simulink library "commdigpbndpm2"  (Simulink 5.0)
undefined symbols (not defined in the file or in its folder): D
libraries: commblksprivate x12, dspsigattribs x6, commdigbbndpm2 x6, dspsigops x3
settings Model: RequirementInfo=9  CovMetricSettings=d  Creator=tdelve  LastModifiedBy=mmclerno

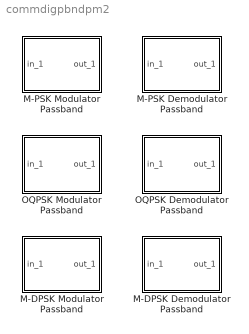
== system commdigpbndpm2 ==
  M-DPSK Demodulator Passband : Subsystem  mask(M-DPSK Demodulator Passband){M=8, OutType=Integer, Dec=Binary, td=1/100, numSamp=1, Fc=3000, Ph=pi/8, InSamp=1/8000}
      mask prompts: M "M-ary number:"; OutType "Output type:"; Dec "Constellation ordering:"; td "Symbol periodl (s):"; numSamp "Baseband samples per symbol:"; Fc "Carrier frequency (Hz):"; Ph "Carrier initial phase (rad):"; InSamp "Input sample time (s):"
      mask help:
      | Demodulate the input signal using the differential phase shift keying method.
      |
      | The input signal must be a sample-based scalar. In case of bit output, the width of the output is the number of bits per symbol. The symbols can be either binary-demapped or Gray-demapped into bits.
      mask init:
      | commblkdyampmdemod('M-DPSK Demodulator Baseband','update');
      | commblkpbndpskmod(gcb,'init');
      mask Help: helpview(commbhelp)
      mask StyleString: edit,popup(Bit|Integer),popup(Binary|Gray),edit,edit,edit,edit,edit
      mask CallbackString: |commblkpbndpskmod(gcb,'InType');||||||
      mask Display:
      | plot(0,0,100,100,[5+1.5*[[0:.8:10] [10:1.6:20] [20:.8:30]] 50 50 50 50+15*[0 1 1 2 2 3]],[85+10*[sin([0:.8:10]*pi*2/5) sin([10:1.6:20]*pi/5) sin([20:.8:30]*pi*2/5)] 85 99 75 85+8*[1 1 -1 -1 1 1]]);
      | disp('M-DPSK')
  M-DPSK Modulator Passband : Subsystem  mask(M-DPSK Modulator Passband){M=8, InType=Integer, Enc=Binary, td=1/100, numSamp=1, Fc=3000, Ph=pi/8, OutSamp=1/8000}
      mask prompts: M "M-ary number:"; InType "Input type:"; Enc "Constellation ordering:"; td "Symbol period (s):"; numSamp "Baseband samples per symbol:"; Fc "Carrier frequency (Hz):"; Ph "Carrier initial phase (rad):"; OutSamp "Output sample time (s):"
      mask help:
      | Modulate the input signal using the differential phase shift keying method.
      |
      | The input signal must be sample-based. In case of integer input, the input must be a scalar. In case of bit input, the width of the input must equal the number of bits per symbol. The bits can be either binary-mapped or Gray-mapped into symbols.
      |
      | The input sample time must equal the symbol period.
      mask init:
      | commblkdyampmmod('M-DPSK Modulator Baseband','update');
      | commblkpbndpskmod(gcb,'init');
      mask Help: helpview(commbhelp)
      mask StyleString: edit,popup(Bit|Integer),popup(Binary|Gray),edit,edit,edit,edit,edit
      mask CallbackString: |commblkpbndpskmod(gcb,'InType');||||||
      mask Display:
      | plot(0,0,100,100,[5+15*[0 1 1 2 2 3] 50 50 50 50+1.5*[[0:.8:10] [10:1.6:20] [20:.8:30]]],[85+8*[1 1 -1 -1 1 1] 85 99 75 85+10*[sin([0:.8:10]*pi*2/5) sin([10:1.6:20]*pi/5) sin([20:.8:30]*pi*2/5)]]);
      | disp('M-DPSK')
  M-PSK Demodulator Passband : Subsystem  mask(M-PSK Demodulator Passband){M=8, OutType=Integer, Dec=Binary, td=1/100, numSamp=1, Fc=3000, Ph=pi/8, InSamp=1/8000}
      mask prompts: M "M-ary number:"; OutType "Output type:"; Dec "Constellation ordering:"; td "Symbol period (s):"; numSamp "Baseband samples per symbol:"; Fc "Carrier frequency (Hz):"; Ph "Carrier initial phase (rad):"; InSamp "Input sample time (s):"
      mask help:
      | Demodulate the input signal using the phase shift keying method.
      |
      | The input signal must be a sample-based scalar. In case of bit output, the width of the output is the number of bits per symbol. The symbols can be either binary-demapped or Gray-demapped into bits.
      mask init:
      | commblkdyampmdemod('M-PSK Demodulator Baseband','update');
      | commblkpbndpskmod(gcb,'init');
      mask Help: helpview(commbhelp)
      mask StyleString: edit,popup(Bit|Integer),popup(Binary|Gray),edit,edit,edit,edit,edit
      mask CallbackString: |commblkpbndpskmod(gcb,'InType');||||||
      mask Display:
      | plot(0,0,100,100,[5+1.5*[[0:.8:10] [10:1.6:20] [20:.8:30]] 50 50 50 50+15*[0 1 1 2 2 3]],[85+10*[sin([0:.8:10]*pi*2/5) sin([10:1.6:20]*pi/5) sin([20:.8:30]*pi*2/5)] 85 99 75 85+8*[1 1 -1 -1 1 1]]);
      | disp('M-PSK')
  M-PSK Modulator Passband : Subsystem  mask(M-PSK Modulator Passband){M=8, InType=Integer, Enc=Binary, td=1/100, numSamp=1, Fc=3000, Ph=pi/8, OutSamp=1/8000}
      mask prompts: M "M-ary number:"; InType "Input type:"; Enc "Constellation ordering:"; td "Symbol period (s):"; numSamp "Baseband samples per symbol:"; Fc "Carrier frequency (Hz):"; Ph "Carrier initial phase (rad):"; OutSamp "Output sample time (s):"
      mask help:
      | Modulate the input signal using the phase shift keying method.
      |
      | The input signal must be sample-based. In case of integer input, the input must be a scalar. In case of bit input, the width of the input must equal the number of bits per symbol. The bits can be either binary-mapped or Gray-mapped into symbols.
      |
      | The input sample time must equal the symbol period.
      mask init:
      | commblkdyampmmod('M-PSK Modulator Baseband','update');
      | commblkpbndpskmod(gcb,'init');
      mask Help: helpview(commbhelp)
      mask StyleString: edit,popup(Bit|Integer),popup(Binary|Gray),edit,edit,edit,edit,edit
      mask CallbackString: |commblkpbndpskmod(gcb,'InType');||||||
      mask Display:
      | plot(0,0,100,100,[5+15*[0 1 1 2 2 3] 50 50 50 50+1.5*[[0:.8:10] [10:1.6:20] [20:.8:30]]],[85+8*[1 1 -1 -1 1 1] 85 99 75 85+10*[sin([0:.8:10]*pi*2/5) sin([10:1.6:20]*pi/5) sin([20:.8:30]*pi*2/5)]]);
      | disp('M-PSK')
  OQPSK Demodulator Passband : Subsystem  mask(OQPSK Demodulator Passband){OutType=Integer, td=1/100, numSamp=7, Fc=3000, Ph=0, InSamp=1/10000}
      mask prompts: OutType "Output type:"; td "Symbol period (s):"; numSamp "Baseband samples per symbol:"; Fc "Carrier frequency (Hz):"; Ph "Carrier initial phase (rad):"; InSamp "Input sample time (s):"
      mask help:
      | Demodulate an offset quadrature phase shift keying modulated signal.
      |
      | The input signal must be a sample-based scalar. In case of bit output, the width of the output is two.
      mask init:
      | commblkdyampmdemod('OQPSK Demodulator Baseband','update');
      mask Help: helpview(commbhelp)
      mask StyleString: popup(Bit|Integer),edit,edit,edit,edit,edit
      mask Display:
      | plot(0,0,100,100,[5+1.5*[[0:.8:10] [10:1.6:20] [20:.8:30]] 50 50 50 50+15*[0 1 1 2 2 3]],[85+10*[sin([0:.8:10]*pi*2/5) sin([10:1.6:20]*pi/5) sin([20:.8:30]*pi*2/5)] 85 99 75 85+8*[1 1 -1 -1 1 1]]);
      | disp('OQPSK')
  OQPSK Modulator Passband : Subsystem  mask(OQPSK Modulator Passband){InType=Integer, td=1/100, numSamp=7, Fc=3000, Ph=0, OutSamp=1/10000}
      mask prompts: InType "Input type:"; td "Symbol period (s):"; numSamp "Baseband samples per symbol:"; Fc "Carrier frequency (Hz):"; Ph "Carrier initial phase (rad):"; OutSamp "Output sample time (s):"
      mask help:
      | Modulate the input signal using offset quadrature phase shift keying method.
      |
      | The input signal must be sample-based. In case of integer input, the input must be a scalar. In case of bit input, the width of the input must be two.
      |
      | The input sample time must equal the symbol period.
      mask init:
      | commblkdyampmmod('OQPSK Modulator Baseband','update');
      mask Help: helpview(commbhelp)
      mask StyleString: popup(Bit|Integer),edit,edit,edit,edit,edit
      mask Display:
      | plot(0,0,100,100,[5+15*[0 1 1 2 2 3] 50 50 50 50+1.5*[[0:.8:10] [10:1.6:20] [20:.8:30]]],[85+8*[1 1 -1 -1 1 1] 85 99 75 85+10*[sin([0:.8:10]*pi*2/5) sin([10:1.6:20]*pi/5) sin([20:.8:30]*pi*2/5)]]);
      | disp('OQPSK')

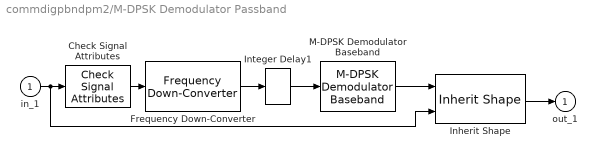
== system commdigpbndpm2/M-DPSK Demodulator Passband ==
  in_1 : Inport
  Check Signal Attributes : dspsigattribs/Check Signal Attributes  SigAttribCheckMethod=Matches attributes exactly  Complexity=Ignore  Frame=Frame-based  DimsCheckMethod=Ignore  Dimensions=1-D  DatatypeCheckMethod=Ignore  DatatypeGeneral=Boolean  DtypeFloatSpecific=Any floating-point  DtypeFixedSpecific=Any fixed-point  DtypeIntSpecific=Any integer  SampleMode=Ignore
  Frequency Down-Converter : commblksprivate/Frequency Down-Converter  Fc=Fc  Ph=Ph  Tin=InSamp  Tout=td/numSamp
  Inherit Shape : commblksprivate/Inherit Shape
  Integer Delay1 : dspsigops/Integer Delay  delay=numSamp-1  ic=0
  M-DPSK Demodulator Baseband : commdigbbndpm2/M-DPSK Demodulator Baseband  M=M  OutType=Integer  Dec=Binary  Ph=0  numSamp=numSamp
  out_1 : Outport  InitialOutput=0
  wires:
  in_1/1 -> Check Signal Attributes/1, Inherit Shape/2
  Check Signal Attributes/1 -> Frequency Down-Converter/1
  Frequency Down-Converter/1 -> Integer Delay1/1
  Integer Delay1/1 -> M-DPSK Demodulator Baseband/1
  M-DPSK Demodulator Baseband/1 -> Inherit Shape/1
  Inherit Shape/1 -> out_1/1

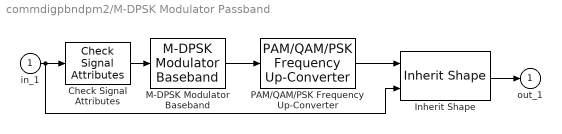
== system commdigpbndpm2/M-DPSK Modulator Passband ==
  in_1 : Inport
  Check Signal Attributes : dspsigattribs/Check Signal Attributes  SigAttribCheckMethod=Matches attributes exactly  Complexity=Ignore  Frame=Frame-based  DimsCheckMethod=Ignore  Dimensions=1-D  DatatypeCheckMethod=Ignore  DatatypeGeneral=Boolean  DtypeFloatSpecific=Any floating-point  DtypeFixedSpecific=Any fixed-point  DtypeIntSpecific=Any integer  SampleMode=Ignore
  Inherit Shape : commblksprivate/Inherit Shape
  M-DPSK Modulator Baseband : commdigbbndpm2/M-DPSK Modulator Baseband  M=M  InType=Integer  Enc=Binary  Ph=0  numSamp=numSamp
  PAM/QAM/PSK Frequency Up-Converter : commblksprivate/PAM//QAM//PSK Frequency Up-Converter  Fc=Fc  Ph=Ph  Tin=td/numSamp  Tout=OutSamp
  out_1 : Outport  InitialOutput=0
  wires:
  in_1/1 -> Check Signal Attributes/1, Inherit Shape/2
  Check Signal Attributes/1 -> M-DPSK Modulator Baseband/1
  M-DPSK Modulator Baseband/1 -> PAM/QAM/PSK Frequency Up-Converter/1
  PAM/QAM/PSK Frequency Up-Converter/1 -> Inherit Shape/1
  Inherit Shape/1 -> out_1/1

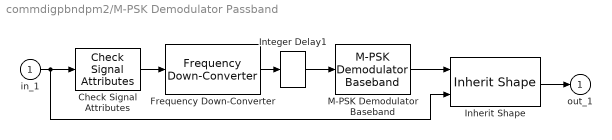
== system commdigpbndpm2/M-PSK Demodulator Passband ==
  in_1 : Inport
  Check Signal Attributes : dspsigattribs/Check Signal Attributes  SigAttribCheckMethod=Matches attributes exactly  Complexity=Ignore  Frame=Frame-based  DimsCheckMethod=Ignore  Dimensions=1-D  DatatypeCheckMethod=Ignore  DatatypeGeneral=Boolean  DtypeFloatSpecific=Any floating-point  DtypeFixedSpecific=Any fixed-point  DtypeIntSpecific=Any integer  SampleMode=Ignore
  Frequency Down-Converter : commblksprivate/Frequency Down-Converter  Fc=Fc  Ph=Ph  Tin=InSamp  Tout=td/numSamp
  Inherit Shape : commblksprivate/Inherit Shape
  Integer Delay1 : dspsigops/Integer Delay  delay=numSamp-1  ic=0
  M-PSK Demodulator Baseband : commdigbbndpm2/M-PSK Demodulator Baseband  M=M  OutType=Integer  Dec=Binary  Ph=0  numSamp=numSamp
  out_1 : Outport  InitialOutput=0
  wires:
  in_1/1 -> Check Signal Attributes/1, Inherit Shape/2
  Check Signal Attributes/1 -> Frequency Down-Converter/1
  Frequency Down-Converter/1 -> Integer Delay1/1
  Integer Delay1/1 -> M-PSK Demodulator Baseband/1
  M-PSK Demodulator Baseband/1 -> Inherit Shape/1
  Inherit Shape/1 -> out_1/1

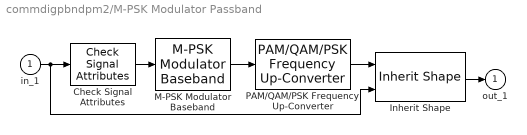
== system commdigpbndpm2/M-PSK Modulator Passband ==
  in_1 : Inport
  Check Signal Attributes : dspsigattribs/Check Signal Attributes  SigAttribCheckMethod=Matches attributes exactly  Complexity=Ignore  Frame=Frame-based  DimsCheckMethod=Ignore  Dimensions=1-D  DatatypeCheckMethod=Ignore  DatatypeGeneral=Boolean  DtypeFloatSpecific=Any floating-point  DtypeFixedSpecific=Any fixed-point  DtypeIntSpecific=Any integer  SampleMode=Ignore
  Inherit Shape : commblksprivate/Inherit Shape
  M-PSK Modulator Baseband : commdigbbndpm2/M-PSK Modulator Baseband  M=M  InType=Integer  Enc=Binary  Ph=0  numSamp=numSamp
  PAM/QAM/PSK Frequency Up-Converter : commblksprivate/PAM//QAM//PSK Frequency Up-Converter  Fc=Fc  Ph=Ph  Tin=td/numSamp  Tout=OutSamp
  out_1 : Outport  InitialOutput=0
  wires:
  in_1/1 -> Inherit Shape/2, Check Signal Attributes/1
  Check Signal Attributes/1 -> M-PSK Modulator Baseband/1
  M-PSK Modulator Baseband/1 -> PAM/QAM/PSK Frequency Up-Converter/1
  PAM/QAM/PSK Frequency Up-Converter/1 -> Inherit Shape/1
  Inherit Shape/1 -> out_1/1

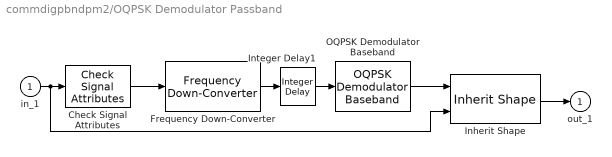
== system commdigpbndpm2/OQPSK Demodulator Passband ==
  in_1 : Inport
  Check Signal Attributes : dspsigattribs/Check Signal Attributes  SigAttribCheckMethod=Matches attributes exactly  Complexity=Ignore  Frame=Frame-based  DimsCheckMethod=Ignore  Dimensions=1-D  DatatypeCheckMethod=Ignore  DatatypeGeneral=Boolean  DtypeFloatSpecific=Any floating-point  DtypeFixedSpecific=Any fixed-point  DtypeIntSpecific=Any integer  SampleMode=Ignore
  Frequency Down-Converter : commblksprivate/Frequency Down-Converter  Fc=Fc  Ph=Ph  Tin=InSamp  Tout=td/(numSamp*2)
  Inherit Shape : commblksprivate/Inherit Shape
  Integer Delay1 : dspsigops/Integer Delay  delay=2*numSamp-1  ic=0
  OQPSK Demodulator Baseband : commdigbbndpm2/OQPSK Demodulator Baseband  OutType=Integer  Ph=0  numSamp=numSamp
  out_1 : Outport  InitialOutput=0
  wires:
  in_1/1 -> Check Signal Attributes/1, Inherit Shape/2
  Frequency Down-Converter/1 -> Integer Delay1/1
  Check Signal Attributes/1 -> Frequency Down-Converter/1
  Integer Delay1/1 -> OQPSK Demodulator Baseband/1
  OQPSK Demodulator Baseband/1 -> Inherit Shape/1
  Inherit Shape/1 -> out_1/1

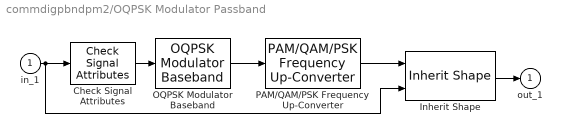
== system commdigpbndpm2/OQPSK Modulator Passband ==
  in_1 : Inport
  Check Signal Attributes : dspsigattribs/Check Signal Attributes  SigAttribCheckMethod=Matches attributes exactly  Complexity=Ignore  Frame=Frame-based  DimsCheckMethod=Ignore  Dimensions=1-D  DatatypeCheckMethod=Ignore  DatatypeGeneral=Boolean  DtypeFloatSpecific=Any floating-point  DtypeFixedSpecific=Any fixed-point  DtypeIntSpecific=Any integer  SampleMode=Ignore
  Inherit Shape : commblksprivate/Inherit Shape
  OQPSK Modulator Baseband : commdigbbndpm2/OQPSK Modulator Baseband  InType=Integer  Ph=0  numSamp=numSamp
  PAM/QAM/PSK Frequency Up-Converter : commblksprivate/PAM//QAM//PSK Frequency Up-Converter  Fc=Fc  Ph=Ph  Tin=td/(numSamp*2)  Tout=OutSamp
  out_1 : Outport  InitialOutput=0
  wires:
  in_1/1 -> Check Signal Attributes/1, Inherit Shape/2
  Check Signal Attributes/1 -> OQPSK Modulator Baseband/1
  OQPSK Modulator Baseband/1 -> PAM/QAM/PSK Frequency Up-Converter/1
  PAM/QAM/PSK Frequency Up-Converter/1 -> Inherit Shape/1
  Inherit Shape/1 -> out_1/1
